simulink model "flightControlSystem"  (R2023a)
settings: Solver=ode3  StartTime=0  StopTime=TFinal  FixedStep=Ts  RelTol=1e-3  EnableMultiTasking=on
undefined symbols (not defined in the file): codertarget, COG_X, COG_Y, Controller, degree_range1, degree_range2, degree_range3, DiscIntNeverNeededParam, Discrete, Estimator, g, gray, init, num_threshold, prev_degree_range, prev_degree_range2, radius, radius2, ROI_Size, rotation_degree, rotation_degree2, Sensors, straight_threshold, strel, Time, Ts, var_acc_angle_N, var_bias_gyr_N, var_gyro_p_N, Vehicle
libraries: simulink x41, slpidlib x4, ctrlSharedLib x4, sharedtransform x3, visionmorphops x2, visiontransforms x2, visiontextngfix x2, simulink_need_slupdate x1, parrotlib x1, visionanalysis x1
(part 4 of 4)

== matlab function flightControlSystem/Image Processing System/MATLAB Function4 ==
  data: bin_image input; prev_ref input; y output; ref1 input; ref2 input; corner input; flag_corner input; COG_X parameter; COG_Y parameter
function y = fcn(bin_image, prev_ref,ref1,ref2,corner, flag_corner,COG_X, COG_Y)
y = zeros(120,160,3);

for i=1:120
    for j=1:160
        if bin_image(i,j)
            y(i,j,:) = [255 255 255];
        end
    end
end

% C = round([corner(1);corner(2)]);% blue
% P = round([prev_ref(1,1);prev_ref(1,2)]);% yellow
R1 = round([COG_X-ref1(1);ref1(2)+COG_Y]);% red
R2 = round([COG_X-ref2(1);ref2(2)+COG_Y]);% purple
% if flag_corner
%     for i = C(1)-1:C(1)+1
%         for j=C(2)-1:C(2)+1
%             if i>=1 && i<=120 && j>=1 && j<=160
%             y(i,j,:)=[0 0 255]; 
%             end
%         end
%     end
% end
% for i = P(1)-1:P(1)+1
%     for j=P(2)-1:P(2)+1
%         if i>=1 && i<=120 && j>=1 && j<=160
%             y(i,j,:)=[200 200 0]; 
%         end
%     end
% end
for i = R1(1)-1:R1(1)+1
    for j=R1(2)-1:R1(2)+1
        if i>=1 && i<=120 && j>=1 && j<=160
            y(i,j,:)=[255 0 0]; 
        end
    end
end
for i = R2(1)-1:R2(1)+1
    for j=R2(2)-1:R2(2)+1
        if i>=1 && i<=120 && j>=1 && j<=160
            y(i,j,:)=[200 0 200]; 
        end
    end
end

% Drone pos
for i = COG_X-1:COG_X+1
    for j=COG_Y-1:COG_Y+1
        if i>=1 && i<=120 && j>=1 && j<=160 && mod(i+j,2)==0
            y(i,j,:)=[0 0 255]; 
        end
    end
end

== matlab function flightControlSystem/Image Processing System/MATLAB Function5 ==
  data: u input; R output; G output; B output
function [R,G,B] = fcn(u)
R = u(:,:,1);
G = u(:,:,2);
B = u(:,:,3);

== matlab function flightControlSystem/Image Processing System/corner detection1/delete_segment1 ==
  data: bin_image input; seg_image output; COG_X parameter; COG_Y parameter
function seg_image = delete_segment(bin_image,COG_X, COG_Y)
L = bwlabel(bin_image,8);
label = L(COG_X,COG_Y);
if label==0
    label = 1;
end
seg_image = L==label;

== matlab function flightControlSystem/Image Processing System/corner detection1/straight line detector/center_line maker ==
  data: center_lines output; flag_corner output; Theta input; Rho input; cnt input; label input; error output
function [center_lines, flag_corner, error] = fcn(Theta, Rho, cnt, label)
    % cnt에 따라 케이스 나누기
    % cnt = 0일 때 오류 => error = 1;
    % cnt = 1일 때 오류 => error = 1;
    % cnt = 2일 때 flag_corner=0 그리고 center_lines 1개 뽑기
    % cnt = 3일 때 flag_corner=1 그리고 center_lines 1개 뽑기(동일한 theta값 외에 한 직선은 무시하는 알고리즘 필요)
    % cnt = 4일 때 flag_corner=1 그리고 center_lines 2개 뽑기
    center_lines = zeros(2,2);
    flag_corner = 0;
    error = 0;
    if cnt == 0 || cnt == 1
        error = 1;
    elseif cnt == 2
        idx1 = find(label==1,1);
        rho1 = Rho(idx1(1));
        theta1 = Theta(idx1(1));
        idx2 = find(label==2,1);
        rho2 = Rho(idx2(1));
        theta2 = Theta(idx2(1));
        if min(abs(theta1 - theta2),180-abs(theta1 - theta2)) <deg2rad(10)
            center_lines(1,1) = (rho1+rho2)/2;
            center_lines(1,2) = (theta1+theta2)/2;
        else
            error = 1;
        end
    elseif cnt == 3
        flag_corner = 1;
        idx1 = find(label==1,1);
        rho1 = Rho(idx1(1));
        theta1 = Theta(idx1(1));
        idx2 = find(label==2,1);
        rho2 = Rho(idx2(1));
        theta2 = Theta(idx2(1));
        idx3 = find(label==3,1);
        rho3 = Rho(idx3(1));
        theta3 = Theta(idx3(1));
        if min(abs(theta1 - theta2),180-abs(theta1 - theta2)) <deg2rad(10)
            center_lines(1,1) = (rho1+rho2)/2;
            center_lines(1,2) = (theta1+theta2)/2;
        elseif min(abs(theta1 - theta3),180-abs(theta1 - theta3)) <deg2rad(10)
            center_lines(1,1) = (rho1+rho3)/2;
            center_lines(1,2) = (theta1+theta3)/2;
        elseif min(abs(theta2 - theta3),180-abs(theta2 - theta3)) <deg2rad(10)
            center_lines(1,1) = (rho2+rho3)/2;
            center_lines(1,2) = (theta2+theta3)/2;
        else
            error = 1;
        end
    elseif cnt == 4
        flag_corner = 1;
        idx1 = find(label==1,1);
        rho1 = Rho(idx1(1));
        theta1 = Theta(idx1(1));
        idx2 = find(label==2,1);
        rho2 = Rho(idx2(1));
        theta2 = Theta(idx2(1));
        idx3 = find(label==3,1);
        rho3 = Rho(idx3(1));
        theta3 = Theta(idx3(1));
        idx4 = find(label==4,1);
        rho4 = Rho(idx4(1));
        theta4 = Theta(idx4(1));
        if min(abs(theta1 - theta2),180-abs(theta1 - theta2)) <deg2rad(10)
            center_lines(1,1) = (rho1+rho2)/2;
            center_lines(1,2) = (theta1+theta2)/2;
            
            center_lines(2,1) = (rho3+rho4)/2;
            center_lines(2,2) = (theta3+theta4)/2;
        elseif min(abs(theta1 - theta3),180-abs(theta1 - theta3)) <deg2rad(10)
            center_lines(1,1) = (rho1+rho3)/2;
            center_lines(1,2) = (theta1+theta3)/2;
        
            center_lines(2,1) = (rho2+rho4)/2;
            center_lines(2,2) = (theta2+theta4)/2;
        elseif min(abs(theta1 - theta4),180-abs(theta1 - theta4)) <deg2rad(10)
            center_lines(1,1) = (rho1+rho4)/2;
            center_lines(1,2) = (theta1+theta4)/2;
            
            center_lines(2,1) = (rho2+rho3)/2;
            center_lines(2,2) = (theta2+theta3)/2;
        else
            error = 1;
        end
    end

== matlab function flightControlSystem/Image Processing System/corner detection1/straight line detector/corner_finder ==
  data: center_Pts input; corner output; cnt input
function corner = fcn(center_Pts,cnt)
corner = zeros(1,2);
if cnt==4
    % Define the points on the first line
    P1 = [center_Pts(1,1) center_Pts(1,2)];
    P2 = [center_Pts(1,3) center_Pts(1,4)];
    % Define the points on the second line
    Q1 = [center_Pts(2,1) center_Pts(2,2)];
    Q2 = [center_Pts(2,3) center_Pts(2,4)];
    if P2(1) - P1(1) == 0 % The first line is vertical
        % Calculate the slope and y-intercept of the second line
        slope_Q = (Q2(2) - Q1(2)) / (Q2(1) - Q1(1));
        y_intercept2 = Q1(2) - slope_Q * Q1(1);

        % Calculate the intersection point
        x_intersect = P1(1);
        y_intersect = slope_Q * x_intersect + y_intercept2;
    elseif Q2(1) - Q1(1) == 0 % The second line is vertical
        % Calculate the slope and y-intercept of the first line
        slope_P = (P2(2) - P1(2)) / (P2(1) - P1(1));
        y_intercept1 = P1(2) - slope_P * P1(1);

        % Calculate the intersection point
        x_intersect = Q1(1);
        y_intersect = slope_P * x_intersect + y_intercept1;
    else % Both lines are not vertical
        % Calculate the slope and y-intercept of each line
        slope_P = (P2(2) - P1(2)) / (P2(1) - P1(1));
        y_intercept1 = P1(2) - slope_P * P1(1);
        slope_Q = (Q2(2) - Q1(2)) / (Q2(1) - Q1(1));
        y_intercept2 = Q1(2) - slope_Q * Q1(1);

        % Calculate the intersection point
        x_intersect = (y_intercept2 - y_intercept1) / (slope_P - slope_Q);
        y_intersect = slope_P * x_intersect + y_intercept1;
    end
    % Output the intersection point
    corner = [y_intersect, x_intersect];
end

== matlab function flightControlSystem/Image Processing System/corner detection1/straight line detector/hough trans of center lines ==
  data: center_lines input; Theta output; Rho output
function [Theta,Rho] = fcn(center_lines)
    Theta = center_lines(:,2);
    Rho = center_lines(:,1);

== matlab function flightControlSystem/Image Processing System/corner detection1/straight line detector/hough trans ==
  data: edge_image input; Theta output; Rho output; cnt output; label output
function [Theta,Rho,cnt,label] = fcn(edge_image)
    [H,T,R] = hough(edge_image);
    P = houghpeaks(H,4,'Threshold',0.3*max(H(:)),'NHoodSize',[19 19]);
    Theta = zeros(4,1);
    Rho = zeros(4,1);
    n = size(P,1);
    for i=1:n
        Rho(i) = R(P(i,1));
        Theta(i) = deg2rad(T(P(i,2)));
    end
    cnt = 0; %서로 다른 라인의 개수
    label = zeros(4,1); %같은 라인끼리 묶는 집합
    for i = 1:n
        if label(i)==0
            cnt = cnt + 1;
            label(i) = cnt;
            if i<n
                for j = i+1:n
                    if label(j) == 0 && abs(Rho(i)-Rho(j))<10 && min(180-abs(Theta(i)-Theta(j)),abs(Theta(i)-Theta(j)))<deg2rad(10)
                            label(j) = cnt;
                    end
                end
            end
        end
    end
